simulink model "Bebop_sim_spline_realtime"  (R2018a)
settings: Solver=VariableStepAuto  StartTime=0.0  StopTime=20  FixedStep=.05  MaxStep=1  MinStep=0.08  RelTol=50  AbsTol=50
values from neighbouring files (symbols this model uses):
  flightplan = [dist,0,height,deg2rad(090) ... (first row only)    [compare_cubic_spline_1.m]    (also in initialize_race_realtime.m; initialize_race_realtime_backup_cubic.m; plot_sim.m = [ 4.348, -0.278, height, deg2rad(  0); test_b_spline.m)
  g = 9.81    [initialize_race_no_realtime.m]    (also in initialize_race_realtime.m; initialize_race_realtime_backup_cubic.m; moving_average_rls_own.m = P(i-1)*meas*(lambda+meas*P(i-1)*meas)^-1)
  gates = sim_gates(:,:,1)    [eval_sim.m]    (also in initialize_race_realtime.m = [dist,0,height,deg2rad(110); initialize_race_realtime_backup_cubic.m = [dist,0,height,deg2rad(110); plot_sim.m)
  max_rot_Z = (90)*pi/180    (= 1.57079632679)    [Bebop_sim_init.m]    (also in initialize_race_no_realtime.m = 1.0471975512; initialize_race_realtime.m; initialize_race_realtime_backup_cubic.m; run_batch1.m = list_agility(idx_agility)*max_rot_Z)
  max_theta_X = (40)*pi/180    (= 0.698131700798)    [Bebop_sim_init.m]    (also in initialize_race_no_realtime.m = 0.13962634016; initialize_race_realtime.m = 1.308996939; initialize_race_realtime_backup_cubic.m = 1.308996939; run_batch1.m = list_agility(idx_agility)*max_theta_X)
  max_theta_Y = (40)*pi/180    (= 0.698131700798)    [Bebop_sim_init.m]    (also in initialize_race_no_realtime.m = 0.13962634016; initialize_race_realtime.m = 1.308996939; initialize_race_realtime_backup_cubic.m = 1.308996939; run_batch1.m = list_agility(idx_agility)*max_theta_Y)
  max_v_Z = .5    (= 0.5)    [Bebop_sim_init.m]    (also in initialize_race_no_realtime.m = 1; initialize_race_realtime.m = 3; initialize_race_realtime_backup_cubic.m = 3; run_batch1.m = list_agility(idx_agility)*max_v_Z)
undefined symbols (not defined in the file or in its folder): fspecial, gray, Rec, SDTV
libraries: sharedtransform x8, simulink x4, visiontextngfix x4, visiontransforms x3, vrlib x2, visionanalysis x2, visionconversions x2, aerolibutil x1, visionstatistics x1, visionsinks x1
(part 2 of 2)

== system Bebop_sim_spline_realtime/Drone input/Contol algorithm/Create Path Frame/Make Y Vector ==
  Velocity Vector : Inport
  Constant : Constant  Value=0
  Demux : Demux  Outputs=3
  Gain : Gain  Gain=-1
  Make Unit : Subsystem
  Matrix Concatenate : Concatenate  NumInputs=3  Mode=Multidimensional array
  Terminator : Terminator
  Y Vector : Outport
  wires:
  Make Unit/1(Unit Vector) -> Y Vector/1
  Velocity Vector/1 -> Demux/1
  Demux/3 -> Terminator/1
  Demux/2 -> Gain/1
  Gain/1 -> Matrix Concatenate/1
  Demux/1 -> Matrix Concatenate/2
  Constant/1 -> Matrix Concatenate/3
  Matrix Concatenate/1 -> Make Unit/1(Vector)

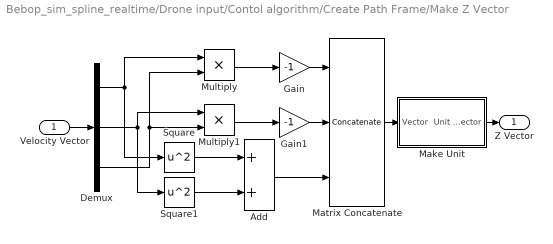
== system Bebop_sim_spline_realtime/Drone input/Contol algorithm/Create Path Frame/Make Z Vector ==
  Velocity Vector : Inport
  Add : Sum
  Demux : Demux  Outputs=3
  Gain : Gain  Gain=-1
  Gain1 : Gain  Gain=-1
  Make Unit : Subsystem
  Matrix Concatenate : Concatenate  NumInputs=3  Mode=Multidimensional array
  Multiply : Product
  Multiply1 : Product
  Square : Math  Operator=square  SaturateOnIntegerOverflow=on
  Square1 : Math  Operator=square  SaturateOnIntegerOverflow=on
  Z Vector : Outport
  wires:
  Make Unit/1(Unit Vector) -> Z Vector/1
  Velocity Vector/1 -> Demux/1
  Demux/3 -> Multiply/2, Multiply1/2
  Matrix Concatenate/1 -> Make Unit/1(Vector)
  Multiply/1 -> Gain/1
  Gain/1 -> Matrix Concatenate/1
  Demux/1 -> Square/1, Multiply/1
  Multiply1/1 -> Gain1/1
  Gain1/1 -> Matrix Concatenate/2
  Demux/2 -> Square1/1, Multiply1/1
  Add/1 -> Matrix Concatenate/3
  Square/1 -> Add/1
  Square1/1 -> Add/2

== system Bebop_sim_spline_realtime/Drone input/Contol algorithm/Create Path Frame/Make X Vector/Make Unit ==
  Vector : Inport
  Multiply : Product
  Reciprocal Sqrt : Sqrt  Operator=rSqrt  SaturateOnIntegerOverflow=on
  Square : Math  Operator=square  SaturateOnIntegerOverflow=on
  Sum of Elements : Sum  Inputs=+
  Unit Vector : Outport
  wires:
  Reciprocal Sqrt/1 -> Multiply/1
  Vector/1 -> Square/1, Multiply/2
  Square/1 -> Sum of Elements/1
  Multiply/1 -> Unit Vector/1
  Sum of Elements/1 -> Reciprocal Sqrt/1

== system Bebop_sim_spline_realtime/Drone input/Contol algorithm/Create Path Frame/Make Y Vector/Make Unit ==
  Vector : Inport
  Multiply : Product
  Reciprocal Sqrt : Sqrt  Operator=rSqrt  SaturateOnIntegerOverflow=on
  Square : Math  Operator=square  SaturateOnIntegerOverflow=on
  Sum of Elements : Sum  Inputs=+
  Unit Vector : Outport
  wires:
  Reciprocal Sqrt/1 -> Multiply/1
  Vector/1 -> Square/1, Multiply/2
  Square/1 -> Sum of Elements/1
  Multiply/1 -> Unit Vector/1
  Sum of Elements/1 -> Reciprocal Sqrt/1

== system Bebop_sim_spline_realtime/Drone input/Contol algorithm/Create Path Frame/Make Z Vector/Make Unit ==
  Vector : Inport
  Multiply : Product
  Reciprocal Sqrt : Sqrt  Operator=rSqrt  SaturateOnIntegerOverflow=on
  Square : Math  Operator=square  SaturateOnIntegerOverflow=on
  Sum of Elements : Sum  Inputs=+
  Unit Vector : Outport
  wires:
  Reciprocal Sqrt/1 -> Multiply/1
  Vector/1 -> Square/1, Multiply/2
  Square/1 -> Sum of Elements/1
  Multiply/1 -> Unit Vector/1
  Sum of Elements/1 -> Reciprocal Sqrt/1

== matlab function Bebop_sim_spline_realtime/Vision System/calculate corners/calculate corners ==
  data: corners_four output; corners input
function corners_four = calculate_corners(corners)
    
    
    %% get bounding box
    corners = double(corners);
    box=[0,0,0,0];
    box(1) = min(corners(:,1));
    box(2) = max(corners(:,1));
    box(3) = min(corners(:,2));
    box(4) = max(corners(:,2));
    
    corners_box = ([box(1), box(3);
                    box(2), box(3);
                    box(1), box(4);
                    box(2), box(4)]);
                
    corners_four = int32(zeros(4,2));
                
    for m = 1:4
        box = corners_box(m,:);
        multi_box = ones(size(corners,1),1) * box;
        diff = multi_box - corners;
        dist = diff(:,1).^2 + diff(:,2).^2;
        [~,i] = min(dist);
        corners_four(m,:) = corners(i,:);
        corners(i,:)=[];
    end
    
end

== matlab function Bebop_sim_spline_realtime/plot3d ==
  data: drone_vel input; drone_pos input; drone_ori input; WP_vel input; WP_yaw input; WP_pos input; gate_pos_global input; gate_ori_global input; current_spline input; WP_list input
function plot3d(drone_vel, drone_pos, drone_ori, WP_vel, WP_yaw, WP_pos, gate_pos_global, gate_ori_global, current_spline, WP_list)
coder.extrinsic('delete')

children = get(gca, 'children');
delete(children(1:12));

gRb = eul2rotm([drone_ori(3),drone_ori(2),drone_ori(1)]);
length = 1;
x_bebop = gRb*[length;0;0];
y_bebop = gRb*[0;length;0];
z_bebop = gRb*[0;0;length];


plot3(drone_pos(1),drone_pos(2),drone_pos(3),'m.','MarkerSize',7)
plot3(drone_pos(1),drone_pos(2),0,'k.','MarkerSize',5)


% spline
d = (0:0.1:1)';
P0 = current_spline(1,:);
P1 = current_spline(2,:);
P2 = current_spline(3,:);
spline_pos = (1-d)*[1,1,1].*((1-d)*P0+d*P1)+d*[1,1,1].*((1-d)*P1 + d*P2);
plot3(spline_pos(:,1),spline_pos(:,2),spline_pos(:,3),'-y','LineWidth',2)


% drone pos
plot3(drone_pos(1)+[0 drone_vel(1)],drone_pos(2)+[0 drone_vel(2)],drone_pos(3)+[0 drone_vel(3)],'k-','LineWidth',2)

% drone ori
plot3(drone_pos(1)+[0 x_bebop(1)],drone_pos(2)+[0 x_bebop(2)],drone_pos(3)+[0 x_bebop(3)],'r-')
plot3(drone_pos(1)+[0 y_bebop(1)],drone_pos(2)+[0 y_bebop(2)],drone_pos(3)+[0 y_bebop(3)],'g-')
plot3(drone_pos(1)+[0 z_bebop(1)],drone_pos(2)+[0 z_bebop(2)],drone_pos(3)+[0 z_bebop(3)],'b-')

% nav pt pos, vel, yaw
plot3(WP_pos(1),WP_pos(2),WP_pos(3),'kx','MarkerSize',10)
plot3(WP_pos(1)+[0 WP_vel(1)],WP_pos(2)+[0 WP_vel(2)],WP_pos(3)+[0 WP_vel(3)],'b-','LineWidth',2)
plot3(WP_pos(1)+[0 0.5*cos(WP_yaw)],WP_pos(2)+[0 0.5*sin(WP_yaw)],WP_pos(3)+[0 0],'r-','LineWidth',1)

% WP current pos
plot3(gate_pos_global(1), gate_pos_global(2), gate_pos_global(3),'kx','LineWidth',2)

% WP current ori
gate_rot = eul2rotm(gate_ori_global);
length = 1;
x_gate = gate_rot*[length;0;0];
y_gate = gate_rot*[0;length;0];
z_gate = gate_rot*[0;0;length];
plot3(gate_pos_global(1) + [0 x_gate(1)],gate_pos_global(2) + [0 x_gate(2)],gate_pos_global(3) + [0 x_gate(3)],'r-','LineWidth',1)
plot3(gate_pos_global(1) + [0 y_gate(1)],gate_pos_global(2) + [0 y_gate(2)],gate_pos_global(3) + [0 y_gate(3)],'g-','LineWidth',1)
plot3(gate_pos_global(1) + [0 z_gate(1)],gate_pos_global(2) + [0 z_gate(2)],gate_pos_global(3) + [0 z_gate(3)],'b-','LineWidth',1)

== matlab function Bebop_sim_spline_realtime/Initialize/reset_plot ==
function reset_plot()
close all;
figure('units','normalized','outerposition',[0 0 0.5 1])
hold on
grid on
axis equal

for i=1:12
    plot3(0,0,0,'m.')
end

% axis([-5,5,-5,5,-2,2])
axis([-5,5,-5,5,0,4])
%view(-20,40) % 3D view
view(-90,90) % top view
%view(-90,0) % front view
xlabel('x')
ylabel('y')
zlabel('z')

== matlab function Bebop_sim_spline_realtime/global2strange drone/MATLAB Function ==
  data: euler input; axang_strange output
function axang_strange = fcn(euler)
m1=zeros(3,3);
m1 = eul2rotm([euler(3),euler(2),euler(1)]);
m2 = eul2rotm([-pi/2, 0, pi/2]);

axang_strange = rotm2axang(m1*m2);

== matlab function Bebop_sim_spline_realtime/Vision System/calculate_PnP ==
  data: tVec output; corners input; size input; rMat output
function [tVec, rMat] = calculate_PnP(corners, size)
    tVec=zeros(1,3);
    rMat=zeros(3,3);
    
    Resolution = 1.5*[320, 200];
    vertFOV = 1.05;
    f = 0.5*Resolution(2)/tan(0.5*vertFOV);
    IntrinsicMatrix = [f, 0, 0;
        0, f, 0;
        Resolution/2, 1];
    cameraParams = cameraParameters('IntrinsicMatrix',IntrinsicMatrix); 
    
    %% calculate extrinsics
    worldPoints = size/2*[1 1;
        1 -1;
        -1 1;
        -1 -1];
    
    corners=double(corners);
    if corners == zeros(4,2)
        disp('no corners')
        return
    end
    
    angles = zeros(6,1);
    k = 1;
    for m=1:3
        for n=m+1:4
            angles(k)=atan2(corners(m,2)-corners(n,2),corners(m,1)-corners(n,1));
            k = k+1;            
        end
    end
    
%     angles(angles<=0) = angles(angles<=0)+pi;
%     
%     a = zeros(2,1);
%     a = hist(angles,unique(angles));
%     if max(a)>2
%         disp('three occurences')
%         return
%     end
%     
%     
%     

    % check how much it resembles rectangle
    if abs(max(corners(:,1))-min(corners(:,1))) < 5
        disp('no rectangle 1')
        corners
        return
    elseif abs(max(corners(:,2))-min(corners(:,2))) < 5
        disp('no rectangle 2')
        corners
        return
    end
    
    angles = zeros(2,1);
    angles(1)=atan2(corners(1,2)-corners(4,2),corners(1,1)-corners(4,1));
    angles(2)=atan2(corners(2,2)-corners(3,2),corners(2,1)-corners(3,1));
    angles(angles<=0) = angles(angles<=0)+pi;
    
    if ~(isequal(unique(angles),sort(angles)))
        temp = corners(3,:);
        corners(3,:) = corners(4,:);
        corners(4,:) = temp;
    end
    
    angles(1)=atan2(corners(1,2)-corners(4,2),corners(1,1)-corners(4,1));
    angles(2)=atan2(corners(2,2)-corners(3,2),corners(2,1)-corners(3,1));
    angles(angles<=0) = angles(angles<=0)+pi;
    
    if ~(isequal(unique(angles),sort(angles)))
        disp('still bad after sort')
        corners
        return
    end    
        
    [rMat,tVec] = extrinsics(corners,worldPoints,cameraParams);
%     [orientation,location] = extrinsicsToCameraPose(rMat,tVec);
    
end

== matlab function Bebop_sim_spline_realtime/gate_global ==
  data: drone_pos input; drone_ori input; gate_pos_global output; tVec input; rMat input; gate_ori_global output
function [gate_pos_global, gate_ori_global]  = gate_global(drone_pos, drone_ori, tVec, rMat)

    gate_pos_global = zeros(3,1);
    gate_ori_global = zeros(1,3);
%     drone_rotm = axang2rotm(drone_ori');
%     gate_pos_local = quatrotate(drone_q,gate_pos_cam);
%     gate_pos_local = drone_rotm * gate_pos_cam';
%     gate_pos_global = gate_pos_local + drone_pos';
%     gate_pos_global = gate_pos_local;

if tVec==zeros(1,3)
    disp('gate_global - no corners')
    return
end
    
    %% drone pos
    drone_pos;
    
    %% drone orientation
    dRg = eul2rotm([drone_ori(3),drone_ori(2),drone_ori(1)]);
    
    %% convert gate pos
    % tVec = right down front, drone was front left up
    dRc = eul2rotm([pi/2,-pi/2,0],'ZYX');
    cRd = dRc^-1;
    cRg = dRg*cRd;
    rel= cRg*tVec';
    gate_pos_global = drone_pos + rel;
    
    % rel = -dRs*tvec';
    % gate_pos_global = drone_pos + rel';
    
    %% convert gate orientation
    rot = squeeze(rMat);
    extra = eul2rotm([0,pi/2,0],'ZYX');
    gate_rot = dRg*cRd*rot^-1*extra;
    gate_ori_global = rotm2eul(gate_rot);
%     
%     wRc = rMat;
%     one_more = 1;%eul2rotm([pi,0,-pi/2]);
%     another_one = 1;%eul2rotm([pi/2,0,0]);
%     wRs = another_one*one_more*cRg*wRc;
%     
%     gate_ori_global = (rotm2eul(wRs))';

     gate_yaw = zeros(1,3);
%       rot = rMat*cRg^-1;
%       gate_yaw=rotm2eul(rot);
    
end

== matlab function Bebop_sim_spline_realtime/global2strange drone/MATLAB Function1 ==
  data: axang output; q input
function axang = fcn(q)

axang = zeros(4,1);

angle = 2 * acos(q(1));
x = q(2) / sqrt(1-q(1)*q(1));
y = q(3) / sqrt(1-q(1)*q(1));
z = q(4) / sqrt(1-q(1)*q(1));

axang(1) = x;
axang(2) = y;
axang(3) = z;
axang(4) = angle;

== matlab function Bebop_sim_spline_realtime/global2strange gate/MATLAB Function1 ==
  data: axang output; q input
function axang = fcn(q)

axang = zeros(4,1);

angle = 2 * acos(q(1));
x = q(2) / sqrt(1-q(1)*q(1));
y = q(3) / sqrt(1-q(1)*q(1));
z = q(4) / sqrt(1-q(1)*q(1));

axang(1) = x;
axang(2) = y;
axang(3) = z;
axang(4) = angle;

== matlab function Bebop_sim_spline_realtime/calculate trajectory/select_WP ==
  data: WP_average output; WP_list input; state0 input; WP_last output
function [WP_average, WP_last] = select_WP(WP_list, state0)
    WP_average=zeros(1,4);
    WP_last=zeros(1,4);

    WP_average = WP_list(state0+1,:);
    if state0 > 0
        WP_last = WP_list(state0,:);
    else
        WP_last = WP_list(end,:);
    end
end

== matlab function Bebop_sim_spline_realtime/calculate trajectory/create_spline ==
  data: WP_average input; current_spline output; WP_last input
function current_spline = create_spline(WP_average, WP_last)
current_spline = zeros(3,3);

WP1 = WP_last(1:4);
WP2 = WP_average(1:4);
    
%% position
% B(d) = (1-d)[(1-d)P0+dP1]+d[(1-d)P1 + dP2]
% B'(d) = 2(1-d)(P1-P0) + 2d(P2-P1)

% B(0) = P0
% B(1) = P2

P0 = WP1(1:3);
P2 = WP2(1:3);

% g1: WP1(1:3) + m*[cos(WP1(4));sin(WP1(4));0]
% g2: WP2(1:3) - n*[cos(WP2(4));sin(WP2(4));0]

A = [cos(WP1(4)) cos(WP2(4));
     sin(WP1(4)) sin(WP2(4))];
b = -[WP1(1)-WP2(1);
    WP1(2)-WP2(2)];
r = A\b;
m = r(1);
P1 = WP1(1:3) + m*[cos(WP1(4)), sin(WP1(4)), 0];

current_spline = [P0; P1; P2];

%% heading
% B(d) = (1-d)[(1-d)P0+dP1]+d[(1-d)P1 + dP2]
% B'(d) = 2(1-d)(P1-P0) + 2d(P2-P1)

% B(0) = atan2(gates(2,2)-gates(1,2),gates(2,1)-gates(1,1))
% B(1) = gates(2,4)

% P0 = atan2(WP2(2)-WP1(2),WP2(1)-WP1(1));
% P2 = WP2(4);
% unwr = unwrap([P0,P2]);
% P0 = unwr(1);
% P2 = unwr(2);
% 
% m = 0.68;
% P1 = P0 + m*(P2-P0);
% 
% spline = [spline, [P0;P1;P2]];


end

== matlab function Bebop_sim_spline_realtime/calculate trajectory/filter_WP ==
  data: WP_list_out output; state0_out output; WP_list_in input; dist_new input; WP_current_pos input; WP_current_ori input; gates_preflight input; state0_in input
function [WP_list_out, state0_out] = filter_WP(WP_list_in, dist_new, WP_current_pos, WP_current_ori, gates_preflight, state0_in)
    
    WP_list_out = zeros(4,4);

    % initialize waypoints with preflight info
    if isequal(WP_list_in, zeros(4,4))
        disp('start WP')
        WP_list_in = gates_preflight;
    end
   
    % catch state transition
    state0_out = 0;
    state0_out = state0_in;
    if dist_new >= 1
        state0_out = state0_out+1;
        if state0_out == size(WP_list_out,1)
            state0_out = 0;
        end
    end
    
    WP_list_out = WP_list_in;
    
    % check if there is gate information
    if WP_current_ori == zeros(1,3)
        % no gate info
        disp('gate_global - no corners')
        
    else
        % gate info, update WP
        alpha = 0.2;
        
        WP_average = WP_list_out(state0_out+1,:);
        WP_average_pos = WP_average(1:3);
        WP_average_hdg = WP_average(4);
       
        if norm(WP_current_pos' - WP_average_pos) < 0.7
            WP_average_pos = alpha*WP_current_pos' + (1-alpha)*WP_average_pos;
            WP_current_hdg = WP_current_ori(1);
            WP_average_hdg = atan2(alpha*sin(WP_current_hdg) + (1-alpha)*sin(WP_average_hdg), ...
                alpha*cos(WP_current_hdg) + (1-alpha)*cos(WP_average_hdg));
            WP_average = [WP_average_pos, WP_average_hdg];
            WP_list_out(state0_out+1,:) = WP_average;
        end
    end
end

== matlab function Bebop_sim_spline_realtime/Vision System/intersect lines ==
  data: index input; thetas input; corners_output output size=[50,2]; rhos input
function corners_output = intersect_lines(index,thetas,rhos)
% if angle diff is nmore than 45 deg
% then intersect
dist_thresh = 20;

theta=thetas(index(:,1));
rho=rhos(index(:,2));

intersections = zeros(0,2);

for i=1:length(theta)-1
    for j=i+1:length(theta)
        angle_diff = abs(atan2(sin(theta(i)-theta(j)),cos(theta(i)-theta(j))));
        if angle_diff > 40*pi/180 && angle_diff < 140*pi/180
            % intersect lines
            % g1: r1*[cos(t1),sin(t1)] + m*[-sin(t1),cos(t1)]
            % g2: r2*[cos(t2),sin(t2)] + n*[-sin(t2),cos(t2)]
            % equal:
            % r1*cos(t1) - r2*cos(t2) + n*sin(t2) = m*sin(t1) (II in I)
            % r1*sin(t1) - r2*sin(t2) + m*cos(t1) = n*cos(t2)
            % 
            % r1*cos(t1) - r2*cos(t2) + (r1*sin(t1) - r2*sin(t2)))*sin(t2)/cos(t2) = m*(sin(t1) - cos(t1)*sin(t2)/cos(t2))
            ci = cos(theta(i));
            cj = cos(theta(j));
            si = sin(theta(i));
            sj = sin(theta(j));
            ri = rho(i);
            rj = rho(j);
            
            m = (ri*ci-rj*cj+(ri*si-rj*sj)*sj/cj)/(si-ci*sj/cj);
            intersection = ri*[ci,si] + m*[-si,ci];
            
            intersections = [intersections; intersection];
        end
    end    
end

% corners_output = int16(intersections);
% return

clusters = zeros(size(intersections,1),1);
cluster = 0;
corners = zeros(0,2);
votes = zeros(0,1);
while ~all(clusters)
    cluster = cluster+1;
    % find first unclustered and set as center
    s = find(~clusters,1);
    pos_m = intersections(s,:);
    vote_m = 1;
    % set this point as clustered
    clusters(s) = cluster;
    % find points belonging to this cluster until no more were found (and go_around becomes false)
    for i=1:size(intersections,1)
        if ~clusters(i)
            % go through all unclustered points and calculate distance to cluster center
            pos = intersections(i,:);
            distance = norm(pos-pos_m);
            if distance < dist_thresh
                % recalculate average and votes
                pos_m = (pos_m * vote_m + pos) / (vote_m + 1);
                vote_m = vote_m + 1;
                % set point as clustered
                clusters(i) = cluster;
            end
        end
    end
    % finished. add average to a list of clusters
    corners = [corners; pos_m];
    votes = [votes; vote_m];
end

while size(corners,1) > 4
    [~,i]=min(flipud(votes));
    i = size(corners,1) - i + 1;
    corners(i,:)=[];
    votes(i)=[];
end

corners_output = int16(zeros(0,2));
if size(corners,1) == 4
    box=[0,0,0,0];
    box(1) = min(corners(:,1));
    box(2) = max(corners(:,1));
    box(3) = min(corners(:,2));
    box(4) = max(corners(:,2));
    
    corners_box = ([box(1), box(3);
                    box(2), box(3);
                    box(1), box(4);
                    box(2), box(4)]);
           
    
    corners_sorted = zeros(4,2);
    for m = 1:4
        box = corners_box(m,:);
        multi_box = ones(size(corners,1),1) * box;
        diff = multi_box - corners;
        dist = diff(:,1).^2 + diff(:,2).^2;
        [~,i] = min(dist);
        corners_sorted(m,:) = corners(i,:);
        corners(i,:)=[];
    end
    
    corners_output = int16(corners_sorted);
%     corners_output = corners;
end

== matlab function Bebop_sim_spline_realtime/Vision System/calculate_PnP1 ==
  data: tVec output; corners input; size input; rMat output
function [tVec, rMat] = calculate_PnP(corners, size)
    tVec=zeros(1,3);
    rMat=zeros(3,3);
    
    Resolution = 1.5*[320, 200];
    vertFOV = 1.05;
    f = 0.5*Resolution(2)/tan(0.5*vertFOV);
    IntrinsicMatrix = [f, 0, 0;
        0, f, 0;
        Resolution/2, 1];
    cameraParams = cameraParameters('IntrinsicMatrix',IntrinsicMatrix); 
    
    %% calculate extrinsics
    worldPoints = size/2*[1 1;
        1 -1;
        -1 1;
        -1 -1];
    
    corners=double(corners);

    if isempty(corners)
        disp('PnP - no corners')
        return
    end
%     
%     angles = zeros(6,1);
%     k = 1;
%     for m=1:3
%         for n=m+1:4
%             angles(k)=atan2(corners(m,2)-corners(n,2),corners(m,1)-corners(n,1));
%             k = k+1;            
%         end
%     end
%     
% %     angles(angles<=0) = angles(angles<=0)+pi;
% %     
% %     a = zeros(2,1);
% %     a = hist(angles,unique(angles));
% %     if max(a)>2
% %         disp('three occurences')
% %         return
% %     end
% %     
% %     
% %     
% 
%     % check how much it resembles rectangle
%     if abs(max(corners(:,1))-min(corners(:,1))) < 5
%         disp('no rectangle 1')
%         corners
%         return
%     elseif abs(max(corners(:,2))-min(corners(:,2))) < 5
%         disp('no rectangle 2')
%         corners
%         return
%     end
%     
%     angles = zeros(2,1);
%     angles(1)=atan2(corners(1,2)-corners(4,2),corners(1,1)-corners(4,1));
%     angles(2)=atan2(corners(2,2)-corners(3,2),corners(2,1)-corners(3,1));
%     angles(angles<=0) = angles(angles<=0)+pi;
%     
%     if ~(isequal(unique(angles),sort(angles)))
%         temp = corners(3,:);
%         corners(3,:) = corners(4,:);
%         corners(4,:) = temp;
%     end
%     
%     angles(1)=atan2(corners(1,2)-corners(4,2),corners(1,1)-corners(4,1));
%     angles(2)=atan2(corners(2,2)-corners(3,2),corners(2,1)-corners(3,1));
%     angles(angles<=0) = angles(angles<=0)+pi;
%     
%     if ~(isequal(unique(angles),sort(angles)))
%         disp('still bad after sort')
%         corners
%         return
%     end    
        
    [rMat,tVec] = extrinsics(corners,worldPoints,cameraParams);
%     [orientation,location] = extrinsicsToCameraPose(rMat,tVec);
    
end
